simulink model "PVConverter_final"  (R2018a)
settings: Solver=VariableStepAuto  StartTime=0.0  StopTime=43200  RelTol=1e-3
InitFcn:
  | load PVOut_final;
  | Vin = timeseries(ans.Data(:,1),ans.Time);
  | irradiance = 1000;
  | i_ac_ref = 20.05;
  | v_dc_ref = 342;
  | temperature = 20;
  | f_pwm = 10000;
  | L = 0.005;
  | C = 5000e-6;
  | ts = 1/f_pwm/10;
  | v_ac_nom = 220;
  | fbase = 50;
values from neighbouring files (symbols this model uses):
  ans = [0  1; -0.103768511938  1.10376852529]    [PV_model_data.mat]
undefined symbols (not defined in the file or in its folder): CL, DiscIntNeverNeededParam
libraries: powerlib x14
settings Model: Creator=Mehdi  LastModifiedBy=Mehdi

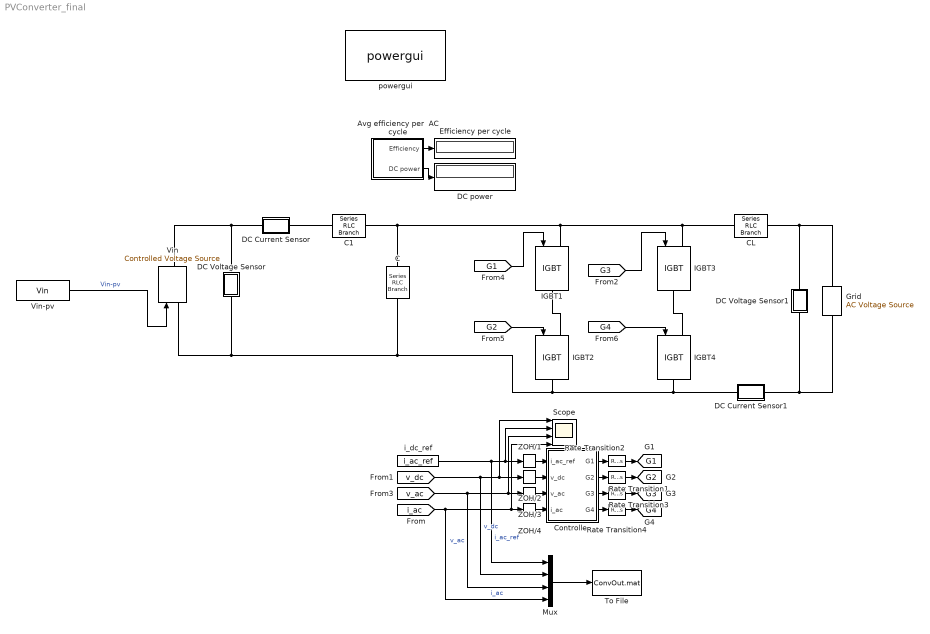
== system PVConverter_final ==
  Avg efficiency per  AC cycle : Subsystem
  C : powerlib/Elements/Series RLC Branch  LConnTagsString=__new0  RConnTagsString=__new0  BranchType=C  Resistance=.04E003  Inductance=0.006  SetiL0=off  InitialCurrent=0  Capacitance=C  Setx0=off  InitialVoltage=0  Measurements=None
  C1 : powerlib/Elements/Series RLC Branch  LConnTagsString=__new0  RConnTagsString=__new0  BranchType=R  Resistance=.04E003  Inductance=0.006  SetiL0=off  InitialCurrent=0  Capacitance=C  Setx0=off  InitialVoltage=0  Measurements=None
  CL : powerlib/Elements/Series RLC Branch  LConnTagsString=__new0  RConnTagsString=__new0  BranchType=L  Resistance=1e-003  Inductance=L  SetiL0=off  InitialCurrent=0  Capacitance=CL  Setx0=off  InitialVoltage=0  Measurements=None
  Controller : Subsystem
  DC Current Sensor : Subsystem
      mask Display: disp('i')
  DC Current Sensor1 : Subsystem
      mask Display: disp('i')
  DC Voltage Sensor : Subsystem
      mask Display: disp('v');
  DC Voltage Sensor1 : Subsystem
      mask Display: disp('v');
  DC power : Display
  Efficiency per cycle : Display
  Grid : powerlib/Electrical Sources/AC Voltage Source  Amplitude=v_ac_nom*sqrt(2)  Phase=0  Frequency=fbase  SampleTime=0  Measurements=None  BusType=swing  Pref=10e3  Qref=0  Qmin=-inf  Qmax=+inf
  IGBT{1..4} (4 alike) : powerlib/Power Electronics/IGBT  Ron=0.001  Lon=0  Vf=1  Tf=1e-6  Tt=2e-6  IC=0  Rs=1e5  Cs=inf  Measurements=off
  Mux : Mux
  Rate Transition{1..4} (4 alike) : RateTransition
  Scope : Scope  NumInputPorts=4
  To File : ToFile  Filename=ConvOut.mat  MatrixName=SigOut  SaveFormat=Timeseries  SampleTime=1/60
  Vin : powerlib/Electrical Sources/Controlled Voltage Source  Initialize=on  Source_Type=AC  Amplitude=0  Phase=0  Frequency=0  Measurements=None
  Vin-pv : FromWorkspace  VariableName=Vin  SampleTime=1
  ZOH/{1..4} (4 alike) : ZeroOrderHold  SampleTime=ts
  i_dc_ref : Constant  Value=i_ac_ref
  powergui : powerlib/powergui  SimulationMode=Discrete  SampleTime=5.0e-4  frequency=60  Iterations=50  frequencyindice=0  Pbase=100e6  ErrMax=1e-4  UnitsV=kV  UnitsW=MW  buscounter=0  FunctionMessages=off  echomessages=off  EnableUseOfTLC=off  CurrentSourceSwitches=off  DisableSnubberDevices=off  DisableRonSwitches=off  DisableVfSwitches=off  DisplayEquations=off  SolverType=Tustin/Backward Euler (TBE)  Interpol=off  ExternalGateDelay=off  methode=off  Ts=100  x0status=blocks  SPID=off  SwTol=0  HookPort=off  RestoreLinks=warning  ResistiveCurrentMeasurement=off  Frange=[0:2:500]  Ylog=off  Xlog=on  ShowGrid=off  save=off  variable=ZData  structure=i_ac  ZoomFFT=off  StartTime=0  cycles=800  DisplayStyle=1  fundamental=50  FreqAxis=off  MaxFrequency=1000  frequencyindicesteady=1  RmsSteady=1  display=off
  tag scope: G1=global, G2=global, G3=global, G4=global
  wires:
  Mux/1 -> To File/1
  i_dc_ref/1 -> Scope/2, ZOH/1/1, Mux/1  "i_ac_ref"
  ZOH/1/1 -> Controller/1(i_ac_ref)
  ZOH/2/1 -> Controller/2(v_dc)
  [i_ac] -> ZOH/4/1, Scope/4, Mux/4  "i_ac"
  [v_ac] -> ZOH/3/1, Scope/3, Mux/3  "v_ac"
  [v_dc] -> Scope/1, ZOH/2/1, Mux/2  "v_dc"
  Rate Transition4/1 -> [G4]
  Controller/4(G4) -> Rate Transition4/1
  Rate Transition3/1 -> [G3]
  Controller/3(G3) -> Rate Transition3/1
  Rate Transition1/1 -> [G2]
  Controller/2(G2) -> Rate Transition1/1
  Rate Transition2/1 -> [G1]
  Controller/1(G1) -> Rate Transition2/1
  ZOH/4/1 -> Controller/4(i_ac)
  ZOH/3/1 -> Controller/3(v_ac)
  [G1] -> IGBT1/1
  [G2] -> IGBT2/1
  [G3] -> IGBT3/1
  [G4] -> IGBT4/1
  Avg efficiency per  AC cycle/2(DC power) -> DC power/1
  Avg efficiency per  AC cycle/1(Efficiency) -> Efficiency per cycle/1
  Vin-pv/1 -> Vin/1  "Vin-pv"
  connections:
  C/RConn1 -- DC Voltage Sensor/LConn1 -- Vin/LConn1 -- DC Current Sensor1/LConn1 -- IGBT4/RConn1 -- IGBT2/RConn1
  C/LConn1 -- C1/RConn1 -- IGBT3/LConn1 -- CL/LConn1 -- IGBT1/LConn1
  IGBT2/LConn1 -- IGBT1/RConn1
  IGBT4/LConn1 -- IGBT3/RConn1
  Grid/RConn1 -- DC Voltage Sensor1/RConn1 -- CL/RConn1
  Grid/LConn1 -- DC Current Sensor1/RConn1 -- DC Voltage Sensor1/LConn1
  DC Voltage Sensor/RConn1 -- DC Current Sensor/RConn1 -- Vin/RConn1
  DC Current Sensor/LConn1 -- C1/LConn1

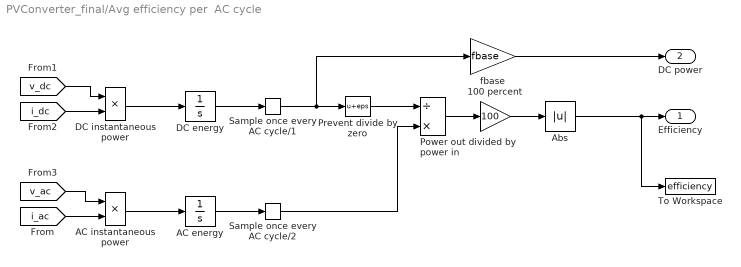
== system PVConverter_final/Avg efficiency per  AC cycle ==
  100 percent : Gain  Gain=100  SaturateOnIntegerOverflow=on  OutDataTypeStr=Inherit: Same as input  ParamDataTypeStr=Inherit: Same as input
  AC energy : Integrator
  AC instantaneous power : Product  SaturateOnIntegerOverflow=on  InputSameDT=on  OutDataTypeStr=Inherit: Same as first input
  Abs : Abs
  DC energy : Integrator
  DC instantaneous power : Product  SaturateOnIntegerOverflow=on  InputSameDT=on  OutDataTypeStr=Inherit: Same as first input
  Power out divided by power in : Product  Inputs=/*  SaturateOnIntegerOverflow=on  InputSameDT=on  OutDataTypeStr=Inherit: Same as first input
  Prevent divide by zero : Bias  Bias=eps
  Sample once every AC cycle/1 : ZeroOrderHold  SampleTime=1/fbase
  Sample once every AC cycle/2 : ZeroOrderHold  SampleTime=1/fbase
  To Workspace : ToWorkspace  VariableName=efficiency  SaveFormat=Structure  SampleTime=-1
      settings: MaxDataPoints=1
  fbase : Gain  Gain=fbase  SaturateOnIntegerOverflow=on  OutDataTypeStr=Inherit: Same as input  ParamDataTypeStr=Inherit: Same as input
  Efficiency : Outport
  DC power : Outport  Port=2
  wires:
  Prevent divide by zero/1 -> Power out divided by power in/1
  DC energy/1 -> Sample once every AC cycle/1/1
  Sample once every AC cycle/1/1 -> fbase/1, Prevent divide by zero/1
  Power out divided by power in/1 -> 100 percent/1
  AC energy/1 -> Sample once every AC cycle/2/1
  AC instantaneous power/1 -> AC energy/1
  DC instantaneous power/1 -> DC energy/1
  [v_ac] -> AC instantaneous power/1
  [i_ac] -> AC instantaneous power/2
  [i_dc] -> DC instantaneous power/2
  [v_dc] -> DC instantaneous power/1
  Sample once every AC cycle/2/1 -> Power out divided by power in/2
  100 percent/1 -> Abs/1
  fbase/1 -> DC power/1
  Abs/1 -> Efficiency/1, To Workspace/1

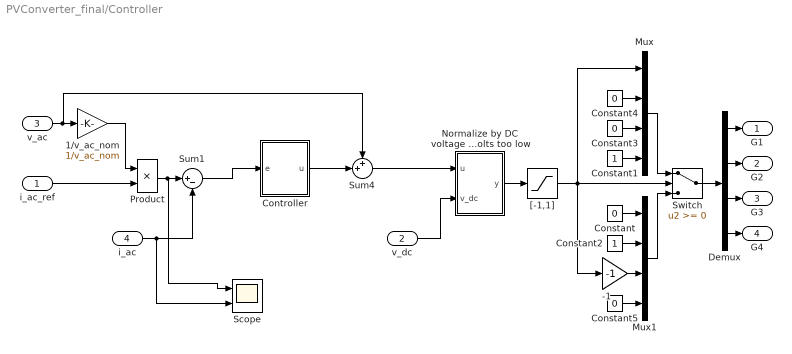
== system PVConverter_final/Controller ==
  i_ac_ref : Inport
  v_dc : Inport  Port=2
  v_ac : Inport  Port=3
  i_ac : Inport  Port=4
  -1 : Gain  Gain=-1  SaturateOnIntegerOverflow=on  OutDataTypeStr=Inherit: Same as input  ParamDataTypeStr=Inherit: Same as input
  1/v_ac_nom : Gain  Gain=1/v_ac_nom  SaturateOnIntegerOverflow=on  OutDataTypeStr=Inherit: Same as input  ParamDataTypeStr=Inherit: Same as input
  Constant{,3..5} (4 alike) : Constant  Value=0
  Constant1 : Constant
  Constant2 : Constant
  Controller : Subsystem
  Demux : Demux
  Mux : Mux
  Mux1 : Mux
  Normalize by DC voltage and disable if DC volts too low : Subsystem
  Product : Product  SaturateOnIntegerOverflow=on  InputSameDT=on  OutDataTypeStr=Inherit: Same as first input
  Scope : Scope  NumInputPorts=2
  Sum1 : Sum  Inputs=|+-  SaturateOnIntegerOverflow=on  InputSameDT=on  OutDataTypeStr=Inherit: Same as first input
  Sum4 : Sum  Inputs=++|  SaturateOnIntegerOverflow=on  InputSameDT=on  OutDataTypeStr=Inherit: Same as first input
  Switch : Switch  InputSameDT=on
  "[-1,1]" : Saturate  UpperLimit=1  LowerLimit=-1
  G1 : Outport
  G2 : Outport  Port=2
  G3 : Outport  Port=3
  G4 : Outport  Port=4
  wires:
  Sum4/1 -> Normalize by DC voltage and disable if DC volts too low/1(u)
  Controller/1(u) -> Sum4/2
  Normalize by DC voltage and disable if DC volts too low/1(y) -> "[-1,1]"/1
  Sum1/1 -> Controller/1(e)
  v_dc/1 -> Normalize by DC voltage and disable if DC volts too low/2(v_dc)
  i_ac_ref/1 -> Product/2
  "[-1,1]"/1 -> Switch/2, Mux/1, -1/1
  Constant2/1 -> Mux1/2
  -1/1 -> Mux1/3
  Constant5/1 -> Mux1/4
  Constant4/1 -> Mux/2
  Constant3/1 -> Mux/3
  Constant1/1 -> Mux/4
  Mux1/1 -> Switch/3
  Constant/1 -> Mux1/1
  Mux/1 -> Switch/1
  Demux/4 -> G4/1
  Demux/3 -> G3/1
  Demux/2 -> G2/1
  Demux/1 -> G1/1
  Switch/1 -> Demux/1
  i_ac/1 -> Scope/2, Sum1/2
  Product/1 -> Scope/1, Sum1/1
  1/v_ac_nom/1 -> Product/1
  v_ac/1 -> 1/v_ac_nom/1, Sum4/1

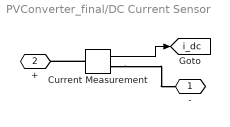
== system PVConverter_final/DC Current Sensor ==
  Current Measurement : powerlib/Measurements/Current Measurement  PhasorSimulation=off  OutputType=Complex  PSBequivalent=0
  - : PMIOPort  Side=Left
  + : PMIOPort  Port=2  Side=Right
  tag scope: i_dc=global
  wires:
  Current Measurement/1 -> [i_dc]
  connections:
  Current Measurement/RConn1 -- -/RConn1
  Current Measurement/LConn1 -- +/RConn1

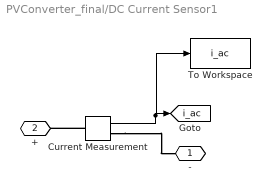
== system PVConverter_final/DC Current Sensor1 ==
  Current Measurement : powerlib/Measurements/Current Measurement  PhasorSimulation=off  OutputType=Complex  PSBequivalent=0
  To Workspace : ToWorkspace  VariableName=i_ac  SaveFormat=Structure With Time  SampleTime=-1
  - : PMIOPort  Side=Left
  + : PMIOPort  Port=2  Side=Right
  tag scope: i_ac=global
  wires:
  Current Measurement/1 -> To Workspace/1, [i_ac]
  connections:
  Current Measurement/LConn1 -- +/RConn1
  Current Measurement/RConn1 -- -/RConn1

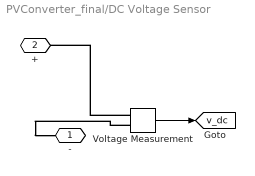
== system PVConverter_final/DC Voltage Sensor ==
  Voltage Measurement : powerlib/Measurements/Voltage Measurement  PhasorSimulation=off  OutputType=Complex  PSBequivalent=0
  - : PMIOPort  Side=Left
  + : PMIOPort  Port=2  Side=Right
  tag scope: v_dc=global
  wires:
  Voltage Measurement/1 -> [v_dc]
  connections:
  Voltage Measurement/LConn2 -- -/RConn1
  Voltage Measurement/LConn1 -- +/RConn1

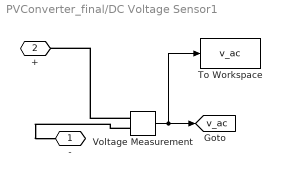
== system PVConverter_final/DC Voltage Sensor1 ==
  To Workspace : ToWorkspace  VariableName=v_ac  SaveFormat=Structure With Time  SampleTime=-1
  Voltage Measurement : powerlib/Measurements/Voltage Measurement  PhasorSimulation=off  OutputType=Complex  PSBequivalent=0
  - : PMIOPort  Side=Left
  + : PMIOPort  Port=2  Side=Right
  tag scope: v_ac=global
  wires:
  Voltage Measurement/1 -> To Workspace/1, [v_ac]
  connections:
  Voltage Measurement/LConn1 -- +/RConn1
  Voltage Measurement/LConn2 -- -/RConn1

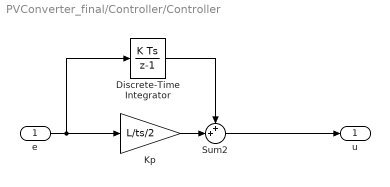
== system PVConverter_final/Controller/Controller ==
  e : Inport
  Discrete-Time Integrator : DiscreteIntegrator  gainval=1000*L/ts  InitialCondition=15  SampleTime=ts  ICPrevOutput=DiscIntNeverNeededParam  ICPrevScaledInput=DiscIntNeverNeededParam
  Kp : Gain  Gain=L/ts/2  SaturateOnIntegerOverflow=on  OutDataTypeStr=Inherit: Same as input  ParamDataTypeStr=Inherit: Same as input
  Sum2 : Sum  Inputs=++|  SaturateOnIntegerOverflow=on  InputSameDT=on  OutDataTypeStr=Inherit: Same as first input
  u : Outport
  wires:
  Discrete-Time Integrator/1 -> Sum2/1
  Sum2/1 -> u/1
  Kp/1 -> Sum2/2
  e/1 -> Kp/1, Discrete-Time Integrator/1

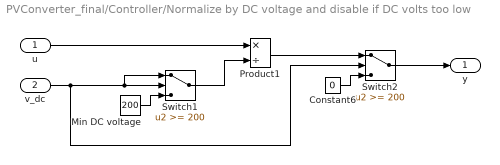
== system PVConverter_final/Controller/Normalize by DC voltage and disable if DC volts too low ==
  u : Inport
  v_dc : Inport  Port=2
  Constant6 : Constant  Value=0
  Min DC voltage : Constant  Value=200
  Product1 : Product  Inputs=*/  SaturateOnIntegerOverflow=on  InputSameDT=on  OutDataTypeStr=Inherit: Same as first input
  Switch1 : Switch  Threshold=200  InputSameDT=on
  Switch2 : Switch  Threshold=200  InputSameDT=on
  y : Outport
  wires:
  Product1/1 -> Switch2/1
  u/1 -> Product1/1
  v_dc/1 -> Switch1/2, Switch1/1, Switch2/2
  Switch2/1 -> y/1
  Switch1/1 -> Product1/2
  Constant6/1 -> Switch2/3
  Min DC voltage/1 -> Switch1/3
